simulink model "regulator_control_1DOF_"  (R2020b)
settings: Solver=VariableStepAuto  StartTime=0.0  StopTime=30  RelTol=1e-3
settings Model: Creator=Admin  LastModifiedBy=Admin

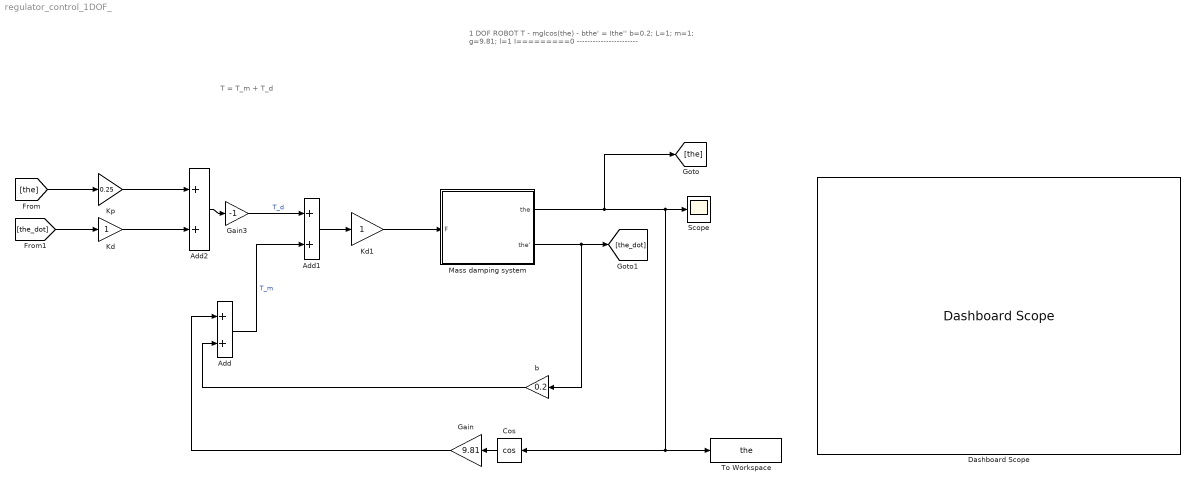
== system regulator_control_1DOF_ ==
  note: T = T_m + T_d
  note: 1 DOF ROBOT
      |
      | T - mglcos(the) - bthe' = Ithe''
      | b=0.2; L=1; m=1; g=9.81; l=1
      |
      | I=========0
      | -----------------------
  Add : Sum
  Add1 : Sum
  Add2 : Sum
  Cos : Trigonometry  Operator=cos
  Dashboard Scope : DashboardScope
  Gain : Gain  Gain=9.81
  Gain3 : Gain  Gain=-1
  Kd : Gain
  Kd1 : Gain
  Kp : Gain  Gain=0.25
  Mass damping system : Subsystem
  Scope : Scope
  To Workspace : ToWorkspace  VariableName=the  SampleTime=-1
  b : Gain  Gain=0.2
  wires:
  Kd1/1 -> Mass damping system/1(F)
  Add1/1 -> Kd1/1
  b/1 -> Add/2
  Mass damping system/1(the) -> Cos/1, To Workspace/1, Scope/1, [the]
  Cos/1 -> Gain/1
  Gain/1 -> Add/1
  Add/1 -> Add1/2  "T_m"
  Add2/1 -> Gain3/1
  Gain3/1 -> Add1/1  "T_d"
  [the] -> Kp/1
  Mass damping system/2(the') -> b/1, [the_dot]
  [the_dot] -> Kd/1
  Kd/1 -> Add2/2
  Kp/1 -> Add2/1

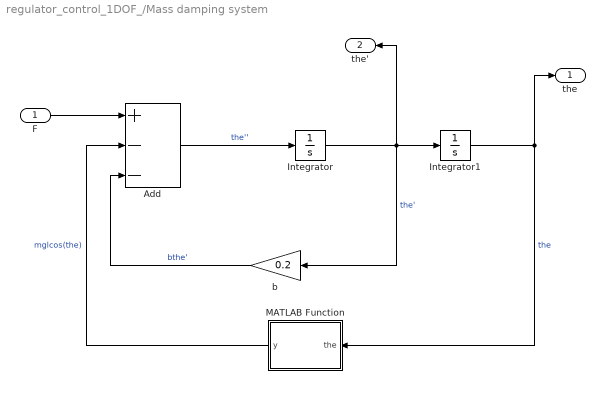
== system regulator_control_1DOF_/Mass damping system ==
  F : Inport
  Add : Sum  Inputs=+--
  Integrator : Integrator
  Integrator1 : Integrator  InitialCondition=pi/4
  MATLAB Function : MATLAB Function  TreatAsAtomicUnit=on
  b : Gain  Gain=0.2
  the : Outport
  the' : Outport  Port=2
  wires:
  Add/1 -> Integrator/1  "the''"
  Integrator1/1 -> MATLAB Function/1(the), the/1  "the"
  Integrator/1 -> the'/1, b/1, Integrator1/1  "the'"
  b/1 -> Add/3  "bthe'"
  MATLAB Function/1(y) -> Add/2  "mglcos(the)"
  F/1 -> Add/1

== matlab function regulator_control_1DOF_/Mass damping system/MATLAB Function ==
  data: the input; y output
function y = fcn(the)

y = 9.81*cos(the);
